simulink model "IM"  (R2022b)
settings: Solver=ode3  StartTime=0.0  StopTime=10.0  FixedStep=1e-5  RelTol=1e-3
libraries: spsIGBTDiodeLib x6, spsCurrentMeasurementLib x3, spsAsynchronousMachineSIUnitsLib x1, spsDCVoltageSourceLib x1, slpidlib x1, simulink x1, sps_lib x1
settings Model: Creator=dhruv  LastModifiedBy=dhruv

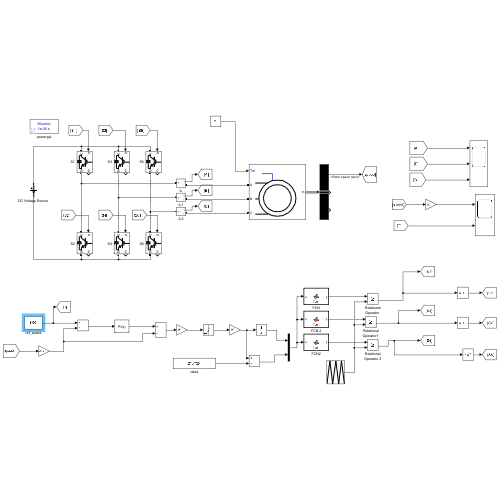
[thumbnail: Simulink's stored preview of the top-level diagram]
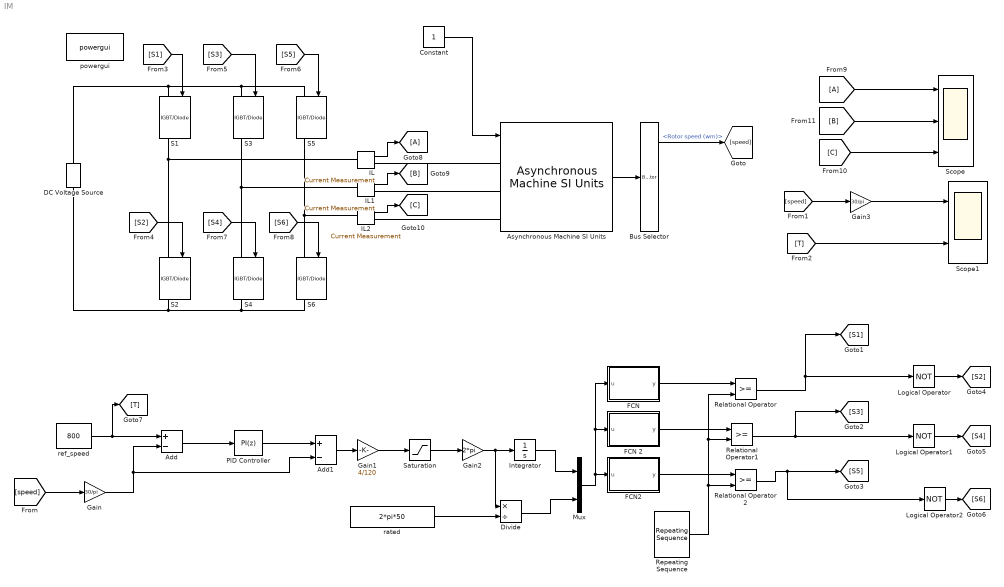
== system IM ==
  Add : Sum  Inputs=+-
  Add1 : Sum  Inputs=+-
  Asynchronous Machine SI Units : spsAsynchronousMachineSIUnitsLib/Asynchronous Machine SI Units  RotorType=Squirrel-cage  PresetModel=No  MechanicalLoad=Torque Tm  ShowDetailedParameters=on  ReferenceFrame=Rotor  Units=SI  MeasurementBus=off  NominalParameters=[1.845e+04 400 50]  VoltageRatio=1  Stator=[0.5968 0.0003495]  Rotor=[0.6258 0.005473]  Cage1=[0.4155 0.002066]  Cage2=[0.4168 0.0003495]  Lm=0.0354  Mechanical=[0.05 0.005879 2]  PolePairs=2  InitialConditions=[0 0 0 0 0 0 0 0]  SimulateSaturation=off  Saturation=[14.03593122, 27.81365428, 53.79336849, 72.68890987, 97.98006896, 148.6815601, 215.7428561, 302.9841135, 428.7778367 ; 230, 322, 414, 460, 506, 552, 598, 644, 690]  LoadFlowParameters=1492000  TsPowergui=0  TsBlock=-1  IterativeModel=Trapezoidal non iterative  IterativeDiscreteModel=Trapezoidal non iterative  Pmec=1.492e+006
  Bus Selector : BusSelector  OutputSignals=Mechanical.Rotor speed (wm),Mechanical.Rotor angle thetam (rad),Mechanical.Electromagnetic torque Te (N*m)
  Constant : Constant
  "DC Voltage Source " : spsDCVoltageSourceLib/DC Voltage Source  Amplitude=650  Measurements=None
  Divide : Product  Inputs=*/
  FCN : MATLAB Function  TreatAsAtomicUnit=on
  FCN 2 : MATLAB Function  TreatAsAtomicUnit=on
  FCN2 : MATLAB Function  TreatAsAtomicUnit=on
  From9 : From
  Gain : Gain  Gain=30/pi
  Gain1 : Gain  Gain=4/120
  Gain2 : Gain  Gain=2*pi
  Gain3 : Gain  Gain=30/pi
  Goto8 : Goto
  IL : spsCurrentMeasurementLib/Current Measurement  PhasorSimulation=off  OutputType=Complex  PSBequivalent=0
  IL1 : spsCurrentMeasurementLib/Current Measurement  PhasorSimulation=off  OutputType=Complex  PSBequivalent=0
  IL2 : spsCurrentMeasurementLib/Current Measurement  PhasorSimulation=off  OutputType=Complex  PSBequivalent=0
  Integrator : Integrator
  Logical Operator : Logic  Operator=NOT  AllPortsSameDT=off  OutDataTypeStr=boolean
  Logical Operator1 : Logic  Operator=NOT  AllPortsSameDT=off  OutDataTypeStr=boolean
  Logical Operator2 : Logic  Operator=NOT  AllPortsSameDT=off  OutDataTypeStr=boolean
  Mux : Mux  Inputs=2
  PID Controller : slpidlib/PID Controller  Controller=PI  Form=Parallel  TimeDomain=Discrete-time  UseExternalTs=off  SampleTime=1e-5  IntegratorMethod=Forward Euler  FilterMethod=Forward Euler  ControllerParametersSource=internal  P=1  I=10  UseKiTs=off  D=0  N=100  UseFilter=on  TunerSelectOption=Transfer Function Based (PID Tuner App)  InitialConditionSource=internal  InitialConditionForIntegrator=0  InitialConditionForFilter=0  DifferentiatorICPrevScaledInput=0  ExternalReset=none  TrackingMode=off  Kt=1  LimitOutput=off  SatLimitsSource=internal  UpperSaturationLimit=inf  LowerSaturationLimit=-inf  LinearizeAsGain=on  AntiWindupMode=none  Kb=1  LimitIntegrator=off  UpperIntegratorSaturationLimit=inf  LowerIntegratorSaturationLimit=-inf  POutMin=[]  POutMax=[]  IOutMin=[]  IOutMax=[]  DOutMin=[]  DOutMax=[]  NOutMin=[]  NOutMax=[]  SumOutMin=[]  SumOutMax=[]  SaturationOutMin=[]  SaturationOutMax=[]  PParamMin=[]  PParamMax=[]  IParamMin=[]  IParamMax=[]  DParamMin=[]  DParamMax=[]  NParamMin=[]  NParamMax=[]  KbParamMin=[]  KbParamMax=[]  KtParamMin=[]  KtParamMax=[]  KbOutMin=[]  KbOutMax=[]  KtOutMin=[]  KtOutMax=[]  IntegratorOutMin=[]  IntegratorOutMax=[]  FilterOutMin=[]  FilterOutMax=[]  SumI1OutMin=[]  SumI1OutMax=[]  SumI2OutMin=[]  SumI2OutMax=[]  SumI3OutMin=[]  SumI3OutMax=[]  SumI4OutMin=[]  SumI4OutMax=[]  SumDOutMin=[]  SumDOutMax=[]  DifferentiatorOutMin=[]  DifferentiatorOutMax=[]  FilterDiffOutCoefMin=[]  FilterDiffOutCoefMax=[]  ReciprocalOutMin=[]  ReciprocalOutMax=[]  SumDenOutMin=[]  SumDenOutMax=[]  SumNumOutMin=[]  SumNumOutMax=[]  DivideOutMin=[]  DivideOutMax=[]  UdiffTsProdOutMin=[]  UdiffTsProdOutMax=[]  NTsProdOutMin=[]  NTsProdOutMax=[]  UintegralTsProdOutMin=[]  UintegralTsProdOutMax=[]  UngainTsProdOutMin=[]  UngainTsProdOutMax=[]  ClampingZeroOutDataTypeStr=Inherit: Inherit via back propagation  ClampingZeroOutMin=[]  ClampingZeroOutMax=[]  FilterDenConstantOutDataTypeStr=Inherit: Inherit via back propagation  FilterDenConstantOutMin=[]  FilterDenConstantOutMax=[]  PCopyOutDataTypeStr=Inherit: Inherit via back propagation  PCopyOutMin=[]  PCopyOutMax=[]  NCopyOutDataTypeStr=Inherit: Inherit via back propagation  NCopyOutMin=[]  NCopyOutMax=[]  IntegratorContinuousStateAttributes=''  IntegratorStateMustResolveToSignalObject=off  IntegratorRTWStateStorageClass=Auto  FilterContinuousStateAttributes=''  FilterStateMustResolveToSignalObject=off  FilterRTWStateStorageClass=Auto  ParallelPVariant=InternalParameters  IdealPVariant=Disabled  IVariant=InternalParameters  DVariant=Disabled  IntegratorVariant=Discrete  SatVariant=Disabled  AWVariant=Passthrough  PCopyVariant=Disabled  TRVariant=Disabled  FdbkBlocksVariant=Forward  IdealPFdbkVariant=Disabled  SatFdbkVariant=Disabled  DerivativeFilterVariant=Disabled  NVariant=Disabled  NCopyVariant=Disabled_SignalSpec  FilterICVariant=Disabled  IntegratorICVariant=InternalICs  ExternalResetVariant=Disabled  TRSumVariant=Passthrough  SumFdbkVariant=Disabled  SumVariant=Sum_PI  TsampFilterVariant=InternalTs  TsampNgainVariant=Passthrough  TsampIntegralVariant=Passthrough  ExternalSaturationOutDataTypeStr=Inherit: Same as second input
  "Relational Operator " : RelationalOperator  OutDataTypeStr=boolean  RndMeth=Simplest  InputSameDT=off
  Relational Operator 2 : RelationalOperator  OutDataTypeStr=boolean  RndMeth=Simplest  InputSameDT=off
  "Relational Operator1 " : RelationalOperator  OutDataTypeStr=boolean  RndMeth=Simplest  InputSameDT=off
  Repeating Sequence : simulink/Sources/Repeating Sequence  rep_seq_t=[0 1 2]*(1/5000)  rep_seq_y=[-1 1 -1]
  S{1..6} (6 alike) : spsIGBTDiodeLib/IGBT//Diode  Ron=1e-3  Rs=1e5  Cs=inf  Measurements=on
  Saturation : Saturate  UpperLimit=50  LowerLimit=0
  Scope : Scope  NumInputPorts=3
  Scope1 : Scope  NumInputPorts=2
  powergui : sps_lib/powergui  Priority=1  SimulationMode=Discrete  SampleTime=1e-5  frequency=60  Iterations=50  frequencyindice=50  Pbase=100e6  ErrMax=1e-4  UnitsV=kV  UnitsW=MW  buscounter=0  FunctionMessages=off  echomessages=off  EnableUseOfTLC=off  CurrentSourceSwitches=off  DisableSnubberDevices=off  DisableRonSwitches=off  DisableVfSwitches=off  DisplayEquations=off  AutomaticDiscreteSolvers=off  SolverType=Tustin  Interpol=off  ExternalGateDelay=off  methode=off  Ts=100  x0status=blocks  SPID=on  SwTol=0  HookPort=off  NonlinearTolerance=1e-4  nMaxIteration=100  ContinueOnMaxIteration=off  RestoreLinks=warning  ResistiveCurrentMeasurement=off  Frange=[0:2:500]  Ylog=off  Xlog=on  ShowGrid=off  save=off  variable=ZData  structure=0  ZoomFFT=off  StartTime=0.0  cycles=1  DisplayStyle=1  fundamental=60  FreqAxis=off  MaxFrequency=1000  frequencyindicesteady=1  RmsSteady=1  display=off
  rated : Constant  Value=2*pi*50
  ref_speed : Constant  Value=800
  wires:
  Constant/1 -> Asynchronous Machine SI Units/1
  Asynchronous Machine SI Units/1 -> Bus Selector/1
  ref_speed/1 -> [T], Add/1
  Bus Selector/1 -> [speed]  "<Rotor speed (wm)>"
  [speed] -> Gain/1
  Gain/1 -> Add1/2, Add/2
  Add/1 -> PID Controller/1
  PID Controller/1 -> Add1/1
  Add1/1 -> Gain1/1
  Gain1/1 -> Saturation/1
  Saturation/1 -> Gain2/1
  Gain2/1 -> Divide/1, Integrator/1
  rated/1 -> Divide/2
  Integrator/1 -> Mux/1
  Divide/1 -> Mux/2
  Mux/1 -> FCN2/1(u), FCN 2/1(u), FCN/1(u)
  FCN/1(y) -> "Relational Operator "/1
  FCN 2/1(y) -> "Relational Operator1 "/1
  FCN2/1(y) -> Relational Operator 2/1
  Repeating Sequence/1 -> "Relational Operator "/2, "Relational Operator1 "/2, Relational Operator 2/2
  "Relational Operator1 "/1 -> [S3], Logical Operator1/1
  Relational Operator 2/1 -> Logical Operator2/1, [S5]
  Logical Operator/1 -> [S2]
  Logical Operator1/1 -> [S4]
  Logical Operator2/1 -> [S6]
  [speed] -> Gain3/1
  Gain3/1 -> Scope1/1
  [T] -> Scope1/2
  [S1] -> S1/1
  [S2] -> S2/1
  [S6] -> S6/1
  [S4] -> S4/1
  [S5] -> S5/1
  [S3] -> S3/1
  IL/1 -> Goto8/1
  IL1/1 -> [B]
  IL2/1 -> [C]
  From9/1 -> Scope/1
  [B] -> Scope/2
  [C] -> Scope/3
  "Relational Operator "/1 -> [S1], Logical Operator/1
  connections:
  S1/LConn1 -- "DC Voltage Source "/RConn1 -- S5/LConn1 -- S3/LConn1
  S1/RConn1 -- S2/LConn1 -- IL/LConn1
  S3/RConn1 -- IL1/LConn1 -- S4/LConn1
  S5/RConn1 -- IL2/LConn1 -- S6/LConn1
  S2/RConn1 -- S6/RConn1 -- S4/RConn1 -- "DC Voltage Source "/LConn1
  IL/RConn1 -- Asynchronous Machine SI Units/LConn1
  IL1/RConn1 -- Asynchronous Machine SI Units/LConn2
  IL2/RConn1 -- Asynchronous Machine SI Units/LConn3

== matlab function IM/FCN ==
  data: u input; y output
function y = fcn(u)
%#codegen

y = u(2)*sin(u(1));

== matlab function IM/FCN2 ==
  data: u input; y output
function y = fcn(u)
%#codegen

y = u(2)*sin(u(1)+(2*pi/3));

== matlab function IM/FCN 2 ==
  data: u input; y output
function y = fcn(u)
%#codegen

y = u(2)*sin(u(1)-(2*pi/3));
